simulink library "NAV420DecodeLib"  (Simulink 7.3)
settings: Solver=ode45  StartTime=0.0  StopTime=10.0  RelTol=1e-3
libraries: NAV420DecodeLib_LowLevel x35
settings Model: Creator=djulzz  LastModifiedBy=djulzz

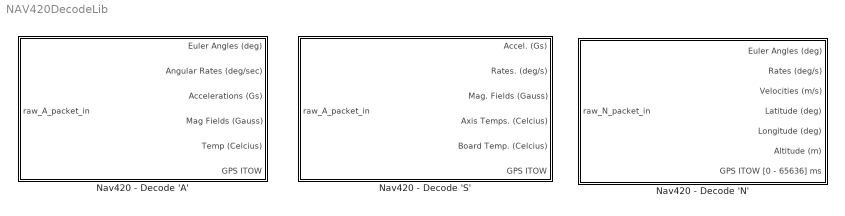
== system NAV420DecodeLib ==
  Nav420 - Decode 'A' : Subsystem
  Nav420 - Decode 'N' : Subsystem
  Nav420 - Decode 'S' : Subsystem

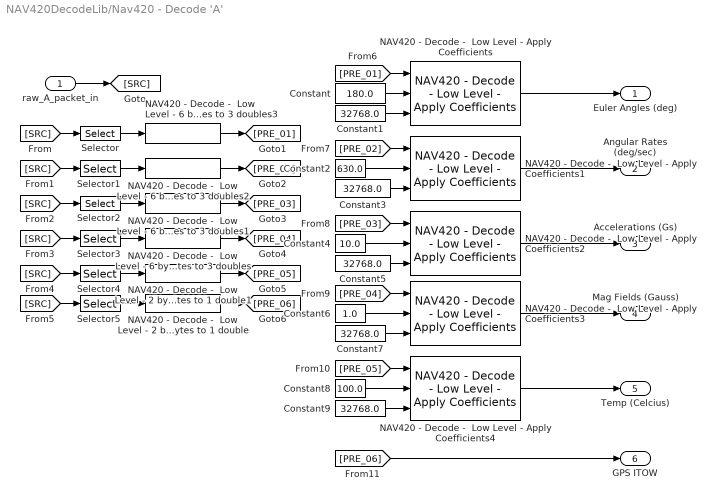
== system NAV420DecodeLib/Nav420 - Decode 'A' ==
  raw_A_packet_in : Inport  DataType=uint8  OutDataType=fixdt(1, 16)  OutScaling=2^0  OutDataTypeStr=uint8
  Constant : Constant  Value=180.0  OutDataTypeMode=double  OutDataType=fixdt(1, 16)  OutScaling=2^0  OutDataTypeStr=double  SampleTime=-1
  Constant{1,3,5,7,9} (5 alike) : Constant  Value=32768.0  OutDataTypeMode=double  OutDataType=fixdt(1, 16)  OutScaling=2^0  OutDataTypeStr=double  SampleTime=-1
  Constant2 : Constant  Value=630.0  OutDataTypeMode=double  OutDataType=fixdt(1, 16)  OutScaling=2^0  OutDataTypeStr=double  SampleTime=-1
  Constant4 : Constant  Value=10.0  OutDataTypeMode=double  OutDataType=fixdt(1, 16)  OutScaling=2^0  OutDataTypeStr=double  SampleTime=-1
  Constant6 : Constant  Value=1.0  OutDataTypeMode=double  OutDataType=fixdt(1, 16)  OutScaling=2^0  OutDataTypeStr=double  SampleTime=-1
  Constant8 : Constant  Value=100.0  OutDataTypeMode=double  OutDataType=fixdt(1, 16)  OutScaling=2^0  OutDataTypeStr=double  SampleTime=-1
  NAV420 - Decode -  Low Level - 2 bytes to 1 double : NAV420DecodeLib_LowLevel/NAV420 - Decode -  Low Level - 2 bytes to 1 double  SystemSampleTime=-1
  NAV420 - Decode -  Low Level - 2 bytes to 1 double1 : NAV420DecodeLib_LowLevel/NAV420 - Decode -  Low Level - 2 bytes to 1 double  SystemSampleTime=-1
  NAV420 - Decode -  Low Level - 6 bytes to 3 doubles{,1..3} (4 alike) : NAV420DecodeLib_LowLevel/NAV420 - Decode -  Low Level - 6 bytes to 3 doubles  SystemSampleTime=-1
  NAV420 - Decode -  Low Level - Apply Coefficients{,1..4} (5 alike) : NAV420DecodeLib_LowLevel/NAV420 - Decode -  Low Level - Apply Coefficients  SystemSampleTime=-1
  Selector : Selector  InputPortWidth=35  IndexOptions=Index vector (dialog)  Indices=[4 5 6 7 8 9]  OutputSizes=1
  Selector1 : Selector  InputPortWidth=35  IndexOptions=Index vector (dialog)  Indices=[10 11 12 13 14 15]  OutputSizes=1
  Selector2 : Selector  InputPortWidth=35  IndexOptions=Index vector (dialog)  Indices=[16 17 18 19 20 21]  OutputSizes=1
  Selector3 : Selector  InputPortWidth=35  IndexOptions=Index vector (dialog)  Indices=[22 23 24 25 26 27]  OutputSizes=1
  Selector4 : Selector  InputPortWidth=35  IndexOptions=Index vector (dialog)  Indices=[28 29]  OutputSizes=1
  Selector5 : Selector  InputPortWidth=35  IndexOptions=Index vector (dialog)  Indices=[30 31]  OutputSizes=1
  Euler Angles (deg) : Outport  DataType=double  OutDataType=fixdt(1, 16)  OutScaling=2^0  OutDataTypeStr=double
  Angular Rates (deg/sec) : Outport  Port=2  DataType=double  OutDataType=fixdt(1, 16)  OutScaling=2^0  OutDataTypeStr=double
  Accelerations (Gs) : Outport  Port=3  DataType=double  OutDataType=fixdt(1, 16)  OutScaling=2^0  OutDataTypeStr=double
  Mag Fields (Gauss) : Outport  Port=4  DataType=double  OutDataType=fixdt(1, 16)  OutScaling=2^0  OutDataTypeStr=double
  Temp (Celcius) : Outport  Port=5  DataType=double  OutDataType=fixdt(1, 16)  OutScaling=2^0  OutDataTypeStr=double
  GPS ITOW : Outport  Port=6  DataType=uint16  OutDataType=fixdt(1, 16)  OutScaling=2^0  OutDataTypeStr=uint16
  wires:
  raw_A_packet_in/1 -> [SRC]
  [SRC] -> Selector/1
  [SRC] -> Selector1/1
  [SRC] -> Selector2/1
  [SRC] -> Selector3/1
  [SRC] -> Selector4/1
  [SRC] -> Selector5/1
  Selector5/1 -> NAV420 - Decode -  Low Level - 2 bytes to 1 double/1
  Selector4/1 -> NAV420 - Decode -  Low Level - 2 bytes to 1 double1/1
  Selector/1 -> NAV420 - Decode -  Low Level - 6 bytes to 3 doubles3/1
  Selector1/1 -> NAV420 - Decode -  Low Level - 6 bytes to 3 doubles2/1
  Selector2/1 -> NAV420 - Decode -  Low Level - 6 bytes to 3 doubles1/1
  Selector3/1 -> NAV420 - Decode -  Low Level - 6 bytes to 3 doubles/1
  NAV420 - Decode -  Low Level - 6 bytes to 3 doubles3/1 -> [PRE_01]
  NAV420 - Decode -  Low Level - 6 bytes to 3 doubles2/1 -> [PRE_02]
  NAV420 - Decode -  Low Level - 6 bytes to 3 doubles1/1 -> [PRE_03]
  NAV420 - Decode -  Low Level - 6 bytes to 3 doubles/1 -> [PRE_04]
  NAV420 - Decode -  Low Level - 2 bytes to 1 double1/1 -> [PRE_05]
  NAV420 - Decode -  Low Level - 2 bytes to 1 double/1 -> [PRE_06]
  [PRE_01] -> NAV420 - Decode -  Low Level - Apply Coefficients/1
  Constant/1 -> NAV420 - Decode -  Low Level - Apply Coefficients/2
  Constant1/1 -> NAV420 - Decode -  Low Level - Apply Coefficients/3
  [PRE_02] -> NAV420 - Decode -  Low Level - Apply Coefficients1/1
  [PRE_03] -> NAV420 - Decode -  Low Level - Apply Coefficients2/1
  [PRE_04] -> NAV420 - Decode -  Low Level - Apply Coefficients3/1
  Constant7/1 -> NAV420 - Decode -  Low Level - Apply Coefficients3/3
  Constant5/1 -> NAV420 - Decode -  Low Level - Apply Coefficients2/3
  Constant3/1 -> NAV420 - Decode -  Low Level - Apply Coefficients1/3
  Constant2/1 -> NAV420 - Decode -  Low Level - Apply Coefficients1/2
  Constant4/1 -> NAV420 - Decode -  Low Level - Apply Coefficients2/2
  Constant6/1 -> NAV420 - Decode -  Low Level - Apply Coefficients3/2
  NAV420 - Decode -  Low Level - Apply Coefficients/1 -> Euler Angles (deg)/1
  NAV420 - Decode -  Low Level - Apply Coefficients1/1 -> Angular Rates (deg/sec)/1
  NAV420 - Decode -  Low Level - Apply Coefficients2/1 -> Accelerations (Gs)/1
  NAV420 - Decode -  Low Level - Apply Coefficients3/1 -> Mag Fields (Gauss)/1
  Constant9/1 -> NAV420 - Decode -  Low Level - Apply Coefficients4/3
  Constant8/1 -> NAV420 - Decode -  Low Level - Apply Coefficients4/2
  [PRE_05] -> NAV420 - Decode -  Low Level - Apply Coefficients4/1
  NAV420 - Decode -  Low Level - Apply Coefficients4/1 -> Temp (Celcius)/1
  [PRE_06] -> GPS ITOW/1

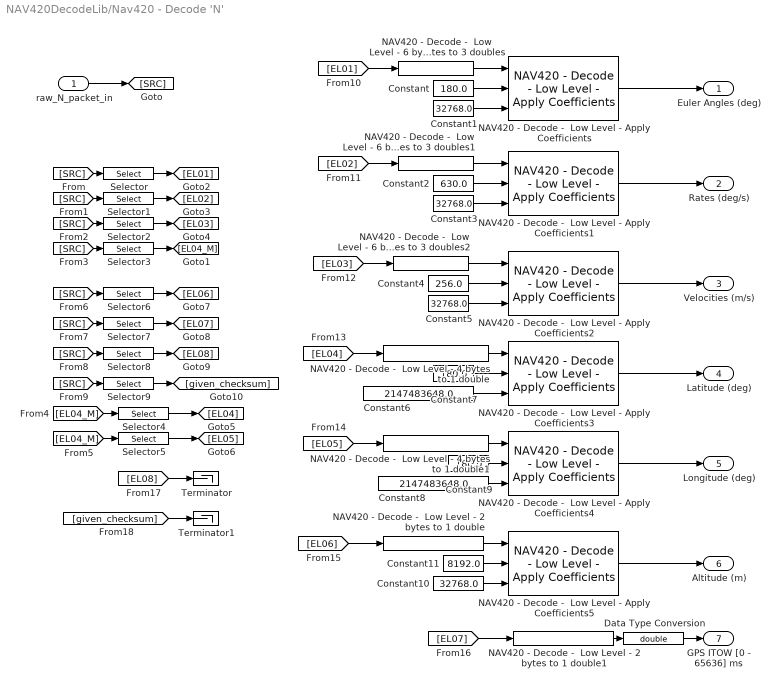
== system NAV420DecodeLib/Nav420 - Decode 'N' ==
  raw_N_packet_in : Inport  DataType=uint8  OutDataType=fixdt(1, 16)  OutScaling=2^0  OutDataTypeStr=uint8
  Constant : Constant  Value=180.0  OutDataTypeMode=double  OutDataType=fixdt(1, 16)  OutScaling=2^0  OutDataTypeStr=double  SampleTime=-1
  Constant{1,3,5,10} (4 alike) : Constant  Value=32768.0  OutDataTypeMode=double  OutDataType=fixdt(1, 16)  OutScaling=2^0  OutDataTypeStr=double  SampleTime=-1
  Constant11 : Constant  Value=8192.0  OutDataTypeMode=double  OutDataType=fixdt(1, 16)  OutScaling=2^0  OutDataTypeStr=double  SampleTime=-1
  Constant2 : Constant  Value=630.0  OutDataTypeMode=double  OutDataType=fixdt(1, 16)  OutScaling=2^0  OutDataTypeStr=double  SampleTime=-1
  Constant4 : Constant  Value=256.0  OutDataTypeMode=double  OutDataType=fixdt(1, 16)  OutScaling=2^0  OutDataTypeStr=double  SampleTime=-1
  Constant6 : Constant  Value=2147483648.0  OutDataTypeMode=double  OutDataType=fixdt(1, 16)  OutScaling=2^0  OutDataTypeStr=double  SampleTime=-1
  Constant7 : Constant  Value=180.0  OutDataTypeMode=double  OutDataType=fixdt(1, 16)  OutScaling=2^0  OutDataTypeStr=double  SampleTime=-1
  Constant8 : Constant  Value=2147483648.0  OutDataTypeMode=double  OutDataType=fixdt(1, 16)  OutScaling=2^0  OutDataTypeStr=double  SampleTime=-1
  Constant9 : Constant  Value=180.0  OutDataTypeMode=double  OutDataType=fixdt(1, 16)  OutScaling=2^0  OutDataTypeStr=double  SampleTime=-1
  Data Type Conversion : DataTypeConversion  OutDataTypeMode=double  OutDataType=fixdt(1, 16)  OutScaling=2^0  OutDataTypeStr=double
  NAV420 - Decode -  Low Level - 2 bytes to 1 double : NAV420DecodeLib_LowLevel/NAV420 - Decode -  Low Level - 2 bytes to 1 double  SystemSampleTime=-1
  NAV420 - Decode -  Low Level - 2 bytes to 1 double1 : NAV420DecodeLib_LowLevel/NAV420 - Decode -  Low Level - 2 bytes to 1 double  SystemSampleTime=-1
  NAV420 - Decode -  Low Level - 4 bytes to 1 double : NAV420DecodeLib_LowLevel/NAV420 - Decode -  Low Level - 4 bytes to 1 double  SystemSampleTime=-1
  NAV420 - Decode -  Low Level - 4 bytes to 1 double1 : NAV420DecodeLib_LowLevel/NAV420 - Decode -  Low Level - 4 bytes to 1 double  SystemSampleTime=-1
  NAV420 - Decode -  Low Level - 6 bytes to 3 doubles : NAV420DecodeLib_LowLevel/NAV420 - Decode -  Low Level - 6 bytes to 3 doubles  SystemSampleTime=-1
  NAV420 - Decode -  Low Level - 6 bytes to 3 doubles1 : NAV420DecodeLib_LowLevel/NAV420 - Decode -  Low Level - 6 bytes to 3 doubles  SystemSampleTime=-1
  NAV420 - Decode -  Low Level - 6 bytes to 3 doubles2 : NAV420DecodeLib_LowLevel/NAV420 - Decode -  Low Level - 6 bytes to 3 doubles  SystemSampleTime=-1
  NAV420 - Decode -  Low Level - Apply Coefficients{,1..5} (6 alike) : NAV420DecodeLib_LowLevel/NAV420 - Decode -  Low Level - Apply Coefficients  SystemSampleTime=-1
  Selector : Selector  InputPortWidth=37  IndexOptions=Index vector (dialog)  Indices=[4 5 6 7 8 9]  OutputSizes=1
  Selector1 : Selector  InputPortWidth=37  IndexOptions=Index vector (dialog)  Indices=[10 11 12 13 14 15]  OutputSizes=1
  Selector2 : Selector  InputPortWidth=37  IndexOptions=Index vector (dialog)  Indices=[16 17 18 19 20 21]  OutputSizes=1
  Selector3 : Selector  InputPortWidth=37  IndexOptions=Index vector (dialog)  Indices=[22 23 24 25 26 27 28 29]  OutputSizes=1
  Selector4 : Selector  InputPortWidth=8  IndexOptions=Index vector (dialog)  Indices=[1 2 3 4]  OutputSizes=1
  Selector5 : Selector  InputPortWidth=8  IndexOptions=Index vector (dialog)  Indices=[5 6 7 8]  OutputSizes=1
  Selector6 : Selector  InputPortWidth=37  IndexOptions=Index vector (dialog)  Indices=[30 31]  OutputSizes=1
  Selector7 : Selector  InputPortWidth=37  IndexOptions=Index vector (dialog)  Indices=[32 33]  OutputSizes=1
  Selector8 : Selector  InputPortWidth=37  IndexOptions=Index vector (dialog)  Indices=[34 35]  OutputSizes=1
  Selector9 : Selector  InputPortWidth=37  IndexOptions=Index vector (dialog)  Indices=[36 37]  OutputSizes=1
  Terminator : Terminator
  Terminator1 : Terminator
  Euler Angles (deg) : Outport  DataType=double  OutDataType=fixdt(1, 16)  OutScaling=2^0  OutDataTypeStr=double
  Rates (deg/s) : Outport  Port=2  DataType=double  OutDataType=fixdt(1, 16)  OutScaling=2^0  OutDataTypeStr=double
  Velocities (m/s) : Outport  Port=3  DataType=double  OutDataType=fixdt(1, 16)  OutScaling=2^0  OutDataTypeStr=double
  Latitude (deg) : Outport  Port=4  DataType=double  OutDataType=fixdt(1, 16)  OutScaling=2^0  OutDataTypeStr=double
  Longitude (deg) : Outport  Port=5  DataType=double  OutDataType=fixdt(1, 16)  OutScaling=2^0  OutDataTypeStr=double
  Altitude (m) : Outport  Port=6  DataType=double  OutDataType=fixdt(1, 16)  OutScaling=2^0  OutDataTypeStr=double
  GPS ITOW [0 - 65636] ms : Outport  Port=7  DataType=double  OutDataType=fixdt(1, 16)  OutScaling=2^0  OutDataTypeStr=double
  wires:
  raw_N_packet_in/1 -> [SRC]
  Selector3/1 -> [EL04_M]
  [EL04_M] -> Selector4/1
  [EL04_M] -> Selector5/1
  Selector4/1 -> [EL04]
  Selector5/1 -> [EL05]
  [SRC] -> Selector/1
  [SRC] -> Selector1/1
  [SRC] -> Selector2/1
  [SRC] -> Selector3/1
  Selector/1 -> [EL01]
  Selector1/1 -> [EL02]
  Selector2/1 -> [EL03]
  Selector6/1 -> [EL06]
  [SRC] -> Selector6/1
  Selector7/1 -> [EL07]
  [SRC] -> Selector7/1
  Selector8/1 -> [EL08]
  [SRC] -> Selector8/1
  Selector9/1 -> [given_checksum]
  [SRC] -> Selector9/1
  [EL08] -> Terminator/1
  [given_checksum] -> Terminator1/1
  [EL01] -> NAV420 - Decode -  Low Level - 6 bytes to 3 doubles/1
  [EL02] -> NAV420 - Decode -  Low Level - 6 bytes to 3 doubles1/1
  [EL03] -> NAV420 - Decode -  Low Level - 6 bytes to 3 doubles2/1
  [EL04] -> NAV420 - Decode -  Low Level - 4 bytes to 1 double/1
  [EL05] -> NAV420 - Decode -  Low Level - 4 bytes to 1 double1/1
  [EL06] -> NAV420 - Decode -  Low Level - 2 bytes to 1 double/1
  [EL07] -> NAV420 - Decode -  Low Level - 2 bytes to 1 double1/1
  NAV420 - Decode -  Low Level - 6 bytes to 3 doubles/1 -> NAV420 - Decode -  Low Level - Apply Coefficients/1
  Constant/1 -> NAV420 - Decode -  Low Level - Apply Coefficients/2
  Constant1/1 -> NAV420 - Decode -  Low Level - Apply Coefficients/3
  NAV420 - Decode -  Low Level - Apply Coefficients/1 -> Euler Angles (deg)/1
  NAV420 - Decode -  Low Level - 6 bytes to 3 doubles1/1 -> NAV420 - Decode -  Low Level - Apply Coefficients1/1
  Constant3/1 -> NAV420 - Decode -  Low Level - Apply Coefficients1/3
  Constant2/1 -> NAV420 - Decode -  Low Level - Apply Coefficients1/2
  NAV420 - Decode -  Low Level - Apply Coefficients1/1 -> Rates (deg/s)/1
  NAV420 - Decode -  Low Level - 6 bytes to 3 doubles2/1 -> NAV420 - Decode -  Low Level - Apply Coefficients2/1
  Constant4/1 -> NAV420 - Decode -  Low Level - Apply Coefficients2/2
  Constant5/1 -> NAV420 - Decode -  Low Level - Apply Coefficients2/3
  NAV420 - Decode -  Low Level - Apply Coefficients2/1 -> Velocities (m/s)/1
  NAV420 - Decode -  Low Level - 4 bytes to 1 double/1 -> NAV420 - Decode -  Low Level - Apply Coefficients3/1
  Constant6/1 -> NAV420 - Decode -  Low Level - Apply Coefficients3/3
  Constant7/1 -> NAV420 - Decode -  Low Level - Apply Coefficients3/2
  NAV420 - Decode -  Low Level - Apply Coefficients3/1 -> Latitude (deg)/1
  NAV420 - Decode -  Low Level - Apply Coefficients4/1 -> Longitude (deg)/1
  NAV420 - Decode -  Low Level - 4 bytes to 1 double1/1 -> NAV420 - Decode -  Low Level - Apply Coefficients4/1
  Constant9/1 -> NAV420 - Decode -  Low Level - Apply Coefficients4/2
  Constant8/1 -> NAV420 - Decode -  Low Level - Apply Coefficients4/3
  NAV420 - Decode -  Low Level - 2 bytes to 1 double/1 -> NAV420 - Decode -  Low Level - Apply Coefficients5/1
  NAV420 - Decode -  Low Level - Apply Coefficients5/1 -> Altitude (m)/1
  Constant11/1 -> NAV420 - Decode -  Low Level - Apply Coefficients5/2
  Constant10/1 -> NAV420 - Decode -  Low Level - Apply Coefficients5/3
  NAV420 - Decode -  Low Level - 2 bytes to 1 double1/1 -> Data Type Conversion/1
  Data Type Conversion/1 -> GPS ITOW [0 - 65636] ms/1

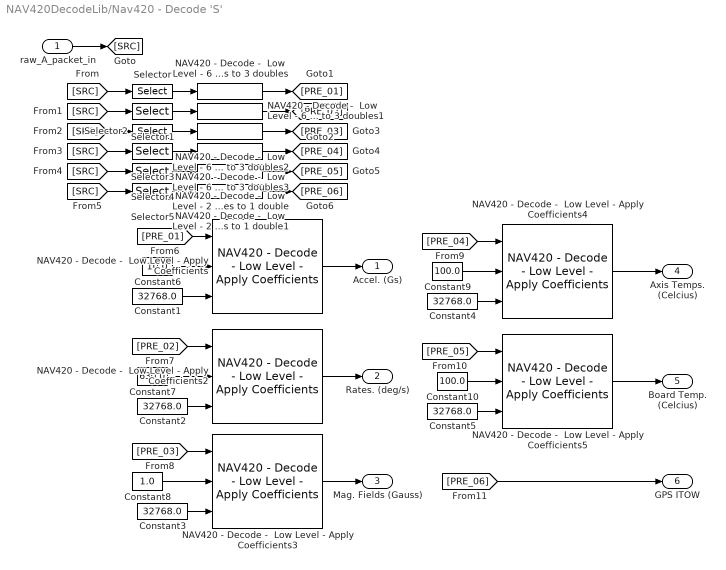
== system NAV420DecodeLib/Nav420 - Decode 'S' ==
  raw_A_packet_in : Inport  DataType=uint8  OutDataType=fixdt(1, 16)  OutScaling=2^0  OutDataTypeStr=uint8
  Constant{1..5} (5 alike) : Constant  Value=32768.0  OutDataTypeMode=double  OutDataType=fixdt(1, 16)  OutScaling=2^0  OutDataTypeStr=double  SampleTime=-1
  Constant10 : Constant  Value=100.0  OutDataTypeMode=double  OutDataType=fixdt(1, 16)  OutScaling=2^0  OutDataTypeStr=double  SampleTime=-1
  Constant6 : Constant  Value=10.0  OutDataTypeMode=double  OutDataType=fixdt(1, 16)  OutScaling=2^0  OutDataTypeStr=double  SampleTime=-1
  Constant7 : Constant  Value=630.0  OutDataTypeMode=double  OutDataType=fixdt(1, 16)  OutScaling=2^0  OutDataTypeStr=double  SampleTime=-1
  Constant8 : Constant  Value=1.0  OutDataTypeMode=double  OutDataType=fixdt(1, 16)  OutScaling=2^0  OutDataTypeStr=double  SampleTime=-1
  Constant9 : Constant  Value=100.0  OutDataTypeMode=double  OutDataType=fixdt(1, 16)  OutScaling=2^0  OutDataTypeStr=double  SampleTime=-1
  NAV420 - Decode -  Low Level - 2 bytes to 1 double : NAV420DecodeLib_LowLevel/NAV420 - Decode -  Low Level - 2 bytes to 1 double  SystemSampleTime=-1
  NAV420 - Decode -  Low Level - 2 bytes to 1 double1 : NAV420DecodeLib_LowLevel/NAV420 - Decode -  Low Level - 2 bytes to 1 double  SystemSampleTime=-1
  NAV420 - Decode -  Low Level - 6 bytes to 3 doubles{,1..3} (4 alike) : NAV420DecodeLib_LowLevel/NAV420 - Decode -  Low Level - 6 bytes to 3 doubles  SystemSampleTime=-1
  NAV420 - Decode -  Low Level - Apply Coefficients{,2..5} (5 alike) : NAV420DecodeLib_LowLevel/NAV420 - Decode -  Low Level - Apply Coefficients  SystemSampleTime=-1
  Selector : Selector  InputPortWidth=35  IndexOptions=Index vector (dialog)  Indices=[4 5 6 7 8 9]  OutputSizes=1
  Selector1 : Selector  InputPortWidth=35  IndexOptions=Index vector (dialog)  Indices=[10 11 12 13 14 15]  OutputSizes=1
  Selector2 : Selector  InputPortWidth=35  IndexOptions=Index vector (dialog)  Indices=[16 17 18 19 20 21]  OutputSizes=1
  Selector3 : Selector  InputPortWidth=35  IndexOptions=Index vector (dialog)  Indices=[22 23 24 25 26 27]  OutputSizes=1
  Selector4 : Selector  InputPortWidth=35  IndexOptions=Index vector (dialog)  Indices=[28 29]  OutputSizes=1
  Selector5 : Selector  InputPortWidth=35  IndexOptions=Index vector (dialog)  Indices=[30 31]  OutputSizes=1
  Accel. (Gs) : Outport  DataType=double  OutDataType=fixdt(1, 16)  OutScaling=2^0  OutDataTypeStr=double
  Rates. (deg/s) : Outport  Port=2  DataType=double  OutDataType=fixdt(1, 16)  OutScaling=2^0  OutDataTypeStr=double
  Mag. Fields (Gauss) : Outport  Port=3  DataType=double  OutDataType=fixdt(1, 16)  OutScaling=2^0  OutDataTypeStr=double
  Axis Temps. (Celcius) : Outport  Port=4  DataType=double  OutDataType=fixdt(1, 16)  OutScaling=2^0  OutDataTypeStr=double
  Board Temp. (Celcius) : Outport  Port=5  DataType=double  OutDataType=fixdt(1, 16)  OutScaling=2^0  OutDataTypeStr=double
  GPS ITOW : Outport  Port=6  DataType=uint16  OutDataType=fixdt(1, 16)  OutScaling=2^0  OutDataTypeStr=uint16
  wires:
  raw_A_packet_in/1 -> [SRC]
  Selector/1 -> NAV420 - Decode -  Low Level - 6 bytes to 3 doubles/1
  Selector1/1 -> NAV420 - Decode -  Low Level - 6 bytes to 3 doubles1/1
  Selector2/1 -> NAV420 - Decode -  Low Level - 6 bytes to 3 doubles2/1
  Selector3/1 -> NAV420 - Decode -  Low Level - 6 bytes to 3 doubles3/1
  [SRC] -> Selector3/1
  [SRC] -> Selector2/1
  [SRC] -> Selector1/1
  [SRC] -> Selector/1
  [SRC] -> Selector4/1
  Selector4/1 -> NAV420 - Decode -  Low Level - 2 bytes to 1 double/1
  [SRC] -> Selector5/1
  Selector5/1 -> NAV420 - Decode -  Low Level - 2 bytes to 1 double1/1
  NAV420 - Decode -  Low Level - 6 bytes to 3 doubles/1 -> [PRE_01]
  NAV420 - Decode -  Low Level - 6 bytes to 3 doubles1/1 -> [PRE_02]
  NAV420 - Decode -  Low Level - 6 bytes to 3 doubles2/1 -> [PRE_03]
  NAV420 - Decode -  Low Level - 6 bytes to 3 doubles3/1 -> [PRE_04]
  NAV420 - Decode -  Low Level - 2 bytes to 1 double/1 -> [PRE_05]
  NAV420 - Decode -  Low Level - 2 bytes to 1 double1/1 -> [PRE_06]
  [PRE_01] -> NAV420 - Decode -  Low Level - Apply Coefficients/1
  [PRE_02] -> NAV420 - Decode -  Low Level - Apply Coefficients2/1
  [PRE_03] -> NAV420 - Decode -  Low Level - Apply Coefficients3/1
  [PRE_04] -> NAV420 - Decode -  Low Level - Apply Coefficients4/1
  [PRE_05] -> NAV420 - Decode -  Low Level - Apply Coefficients5/1
  Constant1/1 -> NAV420 - Decode -  Low Level - Apply Coefficients/3
  Constant2/1 -> NAV420 - Decode -  Low Level - Apply Coefficients2/3
  Constant3/1 -> NAV420 - Decode -  Low Level - Apply Coefficients3/3
  Constant4/1 -> NAV420 - Decode -  Low Level - Apply Coefficients4/3
  Constant5/1 -> NAV420 - Decode -  Low Level - Apply Coefficients5/3
  Constant6/1 -> NAV420 - Decode -  Low Level - Apply Coefficients/2
  Constant7/1 -> NAV420 - Decode -  Low Level - Apply Coefficients2/2
  Constant8/1 -> NAV420 - Decode -  Low Level - Apply Coefficients3/2
  NAV420 - Decode -  Low Level - Apply Coefficients/1 -> Accel. (Gs)/1
  NAV420 - Decode -  Low Level - Apply Coefficients2/1 -> Rates. (deg/s)/1
  NAV420 - Decode -  Low Level - Apply Coefficients3/1 -> Mag. Fields (Gauss)/1
  Constant9/1 -> NAV420 - Decode -  Low Level - Apply Coefficients4/2
  Constant10/1 -> NAV420 - Decode -  Low Level - Apply Coefficients5/2
  [PRE_06] -> GPS ITOW/1
  NAV420 - Decode -  Low Level - Apply Coefficients4/1 -> Axis Temps. (Celcius)/1
  NAV420 - Decode -  Low Level - Apply Coefficients5/1 -> Board Temp. (Celcius)/1
